simulink model "SW_8"  (R2013b)
settings: Solver=ode45  StartTime=0.0  StopTime=128  RelTol=1e-3
values from neighbouring files (symbols this model uses):
  const_val_lenqs = Nq-1    [confSim.m]    (also in preS_confSim.m)
  g = 1    [confSim.m]
  MiS = -5    [confSim.m]
  MS = 5    [confSim.m]
  nb_counter = ceil(log2(Ns))    [confSim.m]    (also in preS_confSim.m)
  NBitsScoreBus = 10    [confSim.m]    (also in preS_confSim.m)
  Nq = length(qCode)    [confSim.m]    (also in preS_confSim.m)
  Ns = length(sCode)    [confSim.m]    (also in preS_confSim.m)
  qCode = base2dec(q,Base)    [confSim.m]
  sCode = base2dec(s,Base)    [confSim.m]
  SMR_len = Nq*3    [confSim.m]    (also in preS_confSim.m)
libraries: xbsIndex_r4 x1212
(part 7 of 7)

== system SW_8/Subsystem/Subsystem4/P1_HW0/Max1 ==
  (i-1,j) : Inport
  (i,j-1) : Inport  Port=2
  (i-1,j-1) : Inport  Port=3
  Concat : xbsIndex_r4/Concat  num_inputs=2  dbl_ovrd=off  block_type=concat
  Constant4 : xbsIndex_r4/Constant  const=0  gui_display_data_type=Fixed-point  arith_type=Unsigned  n_bits=k  bin_pt=kbp  preci_type=Single  exp_width=8  frac_width=24  explicit_period=on  period=Ts  equ=P=C  opselect=C  inp2=PCIN>>17  opr=+  inp1=P  carry=CIN  dbl_ovrd=off  block_type=constant
  Convert1 : xbsIndex_r4/Convert  gui_display_data_type=Fixed-point  arith_type=Unsigned  n_bits=k  bin_pt=0  float_type=Single  exp_bits=8  fraction_bits=24  quantization=Truncate  overflow=Wrap  en=off  latency=c0  dbl_ovrd=off  pipeline=off  block_type=convert
  Convert3 : xbsIndex_r4/Convert  gui_display_data_type=Fixed-point  arith_type=Unsigned  n_bits=NBitsCalcInt  bin_pt=0  float_type=Single  exp_bits=8  fraction_bits=24  quantization=Truncate  overflow=Wrap  en=off  latency=c0  dbl_ovrd=off  pipeline=off  block_type=convert
  Mux : xbsIndex_r4/Mux  inputs=2  en=off  latency=mft  precision=User Defined  arith_type="Signed  (2's comp)"  n_bits=NBitsCalcInt  bin_pt=0  quantization=Truncate  overflow=Wrap  dbl_ovrd=off  block_type=mux
  Mux1 : xbsIndex_r4/Mux  inputs=2  en=off  latency=mft  precision=User Defined  arith_type=Unsigned  n_bits=nb_bool  bin_pt=0  quantization=Truncate  overflow=Wrap  dbl_ovrd=off  block_type=mux
  Mux2 : xbsIndex_r4/Mux  inputs=2  en=off  latency=mft  precision=User Defined  arith_type="Signed  (2's comp)"  n_bits=NBitsCalcInt  bin_pt=0  quantization=Truncate  overflow=Wrap  dbl_ovrd=off  block_type=mux
  Mux6 : xbsIndex_r4/Mux  inputs=2  en=off  latency=mft  precision=User Defined  arith_type="Signed  (2's comp)"  n_bits=NBitsCalcInt  bin_pt=0  quantization=Truncate  overflow=Wrap  dbl_ovrd=off  block_type=mux
  Relational : xbsIndex_r4/Relational  mode=a>b  en=off  latency=r0  dbl_ovrd=off  block_type=relational
  Relational1 : xbsIndex_r4/Relational  mode=a>b  en=off  latency=r0  dbl_ovrd=off  block_type=relational
  Relational3 : xbsIndex_r4/Relational  mode=a>b  en=off  latency=r0  dbl_ovrd=off  block_type=relational
  ind : Outport  InitialOutput=0
  value : Outport  Port=2  InitialOutput=0
  wires:
  Relational/1 -> Mux1/2, Mux/1
  (i-1,j)/1 -> Relational/1, Mux/3
  Constant4/1 -> Mux/2, Relational/2
  Mux/1 -> Mux2/2, Relational1/2  "MS(q_j,s(n))"
  Mux6/1 -> Mux2/3, Relational1/1
  Relational1/1 -> Concat/1, Mux1/1, Mux2/1
  Mux2/1 -> Convert3/1
  Concat/1 -> Convert1/1
  Relational3/1 -> Mux1/3, Mux6/1
  (i,j-1)/1 -> Mux6/3, Relational3/1
  (i-1,j-1)/1 -> Mux6/2, Relational3/2
  Mux1/1 -> Concat/2
  Convert3/1 -> value/1
  Convert1/1 -> ind/1

== system SW_8/Subsystem/Subsystem4/seq_switch/U>U//z ==
  In1 : Inport
  reset : Inport  Port=2
  Convert1 : xbsIndex_r4/Convert  gui_display_data_type=Fixed-point  arith_type=Unsigned  n_bits=nb_bool  bin_pt=0  float_type=Single  exp_bits=8  fraction_bits=24  quantization=Truncate  overflow=Wrap  en=off  latency=c0  dbl_ovrd=off  pipeline=off  block_type=convert
  R_Nq6 : xbsIndex_r4/Register  init=0  rst=on  en=off  dbl_ovrd=off  block_type=register
  Relational2 : xbsIndex_r4/Relational  mode=a>b  en=off  latency=r0  dbl_ovrd=off  block_type=relational
  Out1 : Outport
  wires:
  Convert1/1 -> R_Nq6/1, Relational2/1
  Relational2/1 -> Out1/1
  R_Nq6/1 -> Relational2/2
  In1/1 -> Convert1/1
  reset/1 -> R_Nq6/2

== system SW_8/Subsystem/Subsystem5/Backtracking_final/Subsystem ==
  i(n-1) : Inport
  D(n) : Inport  Port=2
  AddSub : xbsIndex_r4/AddSub  mode=Subtraction  use_carryin=off  use_carryout=off  en=off  latency=as0  precision=User Defined  arith_type=Unsigned  n_bits=NBitsCalcInt  bin_pt=0  quantization=Truncate  overflow=Wrap  dbl_ovrd=off  use_behavioral_HDL=off  hw_selection=Fabric  pipelined=off  block_type=addsub
  Const_0_2 : xbsIndex_r4/Constant  const=0  gui_display_data_type=Fixed-point  arith_type=Unsigned  n_bits=nb_bool  bin_pt=0  preci_type=Single  exp_width=8  frac_width=24  explicit_period=on  period=Ts  equ=P=C  opselect=C  inp2=PCIN>>17  opr=+  inp1=P  carry=CIN  dbl_ovrd=off  block_type=constant
  Const_1_2 : xbsIndex_r4/Constant  const=1  gui_display_data_type=Fixed-point  arith_type=Unsigned  n_bits=1  bin_pt=0  preci_type=Single  exp_width=8  frac_width=24  explicit_period=on  period=Ts  equ=P=C  opselect=C  inp2=PCIN>>17  opr=+  inp1=P  carry=CIN  dbl_ovrd=off  block_type=constant
  Convert1 : xbsIndex_r4/Convert  gui_display_data_type=Fixed-point  arith_type=Unsigned  n_bits=k  bin_pt=0  float_type=Single  exp_bits=8  fraction_bits=24  quantization=Truncate  overflow=Wrap  en=off  latency=c0  dbl_ovrd=off  pipeline=off  block_type=convert
  Convert2 : xbsIndex_r4/Convert  gui_display_data_type=Fixed-point  arith_type=Unsigned  n_bits=counter_num_b  bin_pt=0  float_type=Single  exp_bits=8  fraction_bits=24  quantization=Truncate  overflow=Wrap  en=off  latency=c0  dbl_ovrd=off  pipeline=off  block_type=convert
  Convert3 : xbsIndex_r4/Convert  gui_display_data_type=Fixed-point  arith_type=Unsigned  n_bits=counter_num_b  bin_pt=0  float_type=Single  exp_bits=8  fraction_bits=24  quantization=Truncate  overflow=Wrap  en=off  latency=c0  dbl_ovrd=off  pipeline=off  block_type=convert
  Mux7 : xbsIndex_r4/Mux  inputs=4  en=off  latency=mft  precision=User Defined  arith_type=Unsigned  n_bits=counter_num_b  bin_pt=0  quantization=Truncate  overflow=Wrap  dbl_ovrd=off  block_type=mux
  Mux8 : xbsIndex_r4/Mux  inputs=2  en=off  latency=mft  precision=User Defined  arith_type=Unsigned  n_bits=counter_num_b  bin_pt=0  quantization=Truncate  overflow=Wrap  dbl_ovrd=off  block_type=mux
  Relational2 : xbsIndex_r4/Relational  mode=a<b  en=off  latency=r0  dbl_ovrd=off  block_type=relational
  i(n) : Outport
  StopTBC1 : Outport  Port=2
  wires:
  Convert3/1 -> i(n)/1
  Convert1/1 -> Mux7/1
  Convert2/1 -> Mux7/5, AddSub/1
  Const_1_2/1 -> AddSub/2
  Mux7/1 -> Relational2/1, Mux8/2
  AddSub/1 -> Mux7/3, Mux7/4
  Relational2/1 -> Mux8/1, StopTBC1/1
  Mux8/1 -> Convert3/1
  i(n-1)/1 -> Convert2/1
  D(n)/1 -> Convert1/1
  Const_0_2/1 -> Mux7/2, Relational2/2, Mux8/3

== system SW_8/Subsystem/Subsystem5/Backtracking_final/hi_lo_cast22 ==
  In1 : Inport
  Concat : xbsIndex_r4/Concat  num_inputs=2  dbl_ovrd=off  block_type=concat
  Convert13 : xbsIndex_r4/Convert  gui_display_data_type=Fixed-point  arith_type=Unsigned  n_bits=k  bin_pt=0  float_type=Single  exp_bits=8  fraction_bits=24  quantization=Truncate  overflow=Wrap  en=off  latency=c0  dbl_ovrd=off  pipeline=off  block_type=convert
  Out1 : Outport
  wires:
  In1/1 -> Concat/1, Concat/2
  Concat/1 -> Convert13/1
  Convert13/1 -> Out1/1

== system SW_8/Subsystem/Subsystem5/P1_HW0/Match and Mismtach Score ==
  q_j : Inport
  s(n) : Inport  Port=2
  MS : Inport  Port=3
  MiS : Inport  Port=4
  Mux : xbsIndex_r4/Mux  inputs=2  en=off  latency=mft  precision=User Defined  arith_type="Signed  (2's comp)"  n_bits=NBitsK  bin_pt=0  quantization=Truncate  overflow=Wrap  dbl_ovrd=off  block_type=mux
  Relational : xbsIndex_r4/Relational  mode=a=b  en=off  latency=r0  dbl_ovrd=off  block_type=relational
  MS(q_j,s(n)) : Outport
  wires:
  MiS/1 -> Mux/2
  MS/1 -> Mux/3
  Relational/1 -> Mux/1
  s(n)/1 -> Relational/2
  Mux/1 -> MS(q_j,s(n))/1  "MS(q_j,s(n))"
  q_j/1 -> Relational/1

== system SW_8/Subsystem/Subsystem5/P1_HW0/Max1 ==
  (i-1,j) : Inport
  (i,j-1) : Inport  Port=2
  (i-1,j-1) : Inport  Port=3
  Concat : xbsIndex_r4/Concat  num_inputs=2  dbl_ovrd=off  block_type=concat
  Constant4 : xbsIndex_r4/Constant  const=0  gui_display_data_type=Fixed-point  arith_type=Unsigned  n_bits=k  bin_pt=kbp  preci_type=Single  exp_width=8  frac_width=24  explicit_period=on  period=Ts  equ=P=C  opselect=C  inp2=PCIN>>17  opr=+  inp1=P  carry=CIN  dbl_ovrd=off  block_type=constant
  Convert1 : xbsIndex_r4/Convert  gui_display_data_type=Fixed-point  arith_type=Unsigned  n_bits=k  bin_pt=0  float_type=Single  exp_bits=8  fraction_bits=24  quantization=Truncate  overflow=Wrap  en=off  latency=c0  dbl_ovrd=off  pipeline=off  block_type=convert
  Convert3 : xbsIndex_r4/Convert  gui_display_data_type=Fixed-point  arith_type=Unsigned  n_bits=NBitsCalcInt  bin_pt=0  float_type=Single  exp_bits=8  fraction_bits=24  quantization=Truncate  overflow=Wrap  en=off  latency=c0  dbl_ovrd=off  pipeline=off  block_type=convert
  Mux : xbsIndex_r4/Mux  inputs=2  en=off  latency=mft  precision=User Defined  arith_type="Signed  (2's comp)"  n_bits=NBitsCalcInt  bin_pt=0  quantization=Truncate  overflow=Wrap  dbl_ovrd=off  block_type=mux
  Mux1 : xbsIndex_r4/Mux  inputs=2  en=off  latency=mft  precision=User Defined  arith_type=Unsigned  n_bits=nb_bool  bin_pt=0  quantization=Truncate  overflow=Wrap  dbl_ovrd=off  block_type=mux
  Mux2 : xbsIndex_r4/Mux  inputs=2  en=off  latency=mft  precision=User Defined  arith_type="Signed  (2's comp)"  n_bits=NBitsCalcInt  bin_pt=0  quantization=Truncate  overflow=Wrap  dbl_ovrd=off  block_type=mux
  Mux6 : xbsIndex_r4/Mux  inputs=2  en=off  latency=mft  precision=User Defined  arith_type="Signed  (2's comp)"  n_bits=NBitsCalcInt  bin_pt=0  quantization=Truncate  overflow=Wrap  dbl_ovrd=off  block_type=mux
  Relational : xbsIndex_r4/Relational  mode=a>b  en=off  latency=r0  dbl_ovrd=off  block_type=relational
  Relational1 : xbsIndex_r4/Relational  mode=a>b  en=off  latency=r0  dbl_ovrd=off  block_type=relational
  Relational3 : xbsIndex_r4/Relational  mode=a>b  en=off  latency=r0  dbl_ovrd=off  block_type=relational
  ind : Outport  InitialOutput=0
  value : Outport  Port=2  InitialOutput=0
  wires:
  Relational/1 -> Mux1/2, Mux/1
  (i-1,j)/1 -> Relational/1, Mux/3
  Constant4/1 -> Mux/2, Relational/2
  Mux/1 -> Mux2/2, Relational1/2  "MS(q_j,s(n))"
  Mux6/1 -> Mux2/3, Relational1/1
  Relational1/1 -> Concat/1, Mux1/1, Mux2/1
  Mux2/1 -> Convert3/1
  Concat/1 -> Convert1/1
  Relational3/1 -> Mux1/3, Mux6/1
  (i,j-1)/1 -> Mux6/3, Relational3/1
  (i-1,j-1)/1 -> Mux6/2, Relational3/2
  Mux1/1 -> Concat/2
  Convert3/1 -> value/1
  Convert1/1 -> ind/1

== system SW_8/Subsystem/Subsystem5/seq_switch/U>U//z ==
  In1 : Inport
  reset : Inport  Port=2
  Convert1 : xbsIndex_r4/Convert  gui_display_data_type=Fixed-point  arith_type=Unsigned  n_bits=nb_bool  bin_pt=0  float_type=Single  exp_bits=8  fraction_bits=24  quantization=Truncate  overflow=Wrap  en=off  latency=c0  dbl_ovrd=off  pipeline=off  block_type=convert
  R_Nq6 : xbsIndex_r4/Register  init=0  rst=on  en=off  dbl_ovrd=off  block_type=register
  Relational2 : xbsIndex_r4/Relational  mode=a>b  en=off  latency=r0  dbl_ovrd=off  block_type=relational
  Out1 : Outport
  wires:
  Convert1/1 -> R_Nq6/1, Relational2/1
  Relational2/1 -> Out1/1
  R_Nq6/1 -> Relational2/2
  In1/1 -> Convert1/1
  reset/1 -> R_Nq6/2

== system SW_8/Subsystem/Subsystem6/Backtracking_final/Subsystem ==
  i(n-1) : Inport
  D(n) : Inport  Port=2
  AddSub : xbsIndex_r4/AddSub  mode=Subtraction  use_carryin=off  use_carryout=off  en=off  latency=as0  precision=User Defined  arith_type=Unsigned  n_bits=NBitsCalcInt  bin_pt=0  quantization=Truncate  overflow=Wrap  dbl_ovrd=off  use_behavioral_HDL=off  hw_selection=Fabric  pipelined=off  block_type=addsub
  Const_0_2 : xbsIndex_r4/Constant  const=0  gui_display_data_type=Fixed-point  arith_type=Unsigned  n_bits=nb_bool  bin_pt=0  preci_type=Single  exp_width=8  frac_width=24  explicit_period=on  period=Ts  equ=P=C  opselect=C  inp2=PCIN>>17  opr=+  inp1=P  carry=CIN  dbl_ovrd=off  block_type=constant
  Const_1_2 : xbsIndex_r4/Constant  const=1  gui_display_data_type=Fixed-point  arith_type=Unsigned  n_bits=1  bin_pt=0  preci_type=Single  exp_width=8  frac_width=24  explicit_period=on  period=Ts  equ=P=C  opselect=C  inp2=PCIN>>17  opr=+  inp1=P  carry=CIN  dbl_ovrd=off  block_type=constant
  Convert1 : xbsIndex_r4/Convert  gui_display_data_type=Fixed-point  arith_type=Unsigned  n_bits=k  bin_pt=0  float_type=Single  exp_bits=8  fraction_bits=24  quantization=Truncate  overflow=Wrap  en=off  latency=c0  dbl_ovrd=off  pipeline=off  block_type=convert
  Convert2 : xbsIndex_r4/Convert  gui_display_data_type=Fixed-point  arith_type=Unsigned  n_bits=counter_num_b  bin_pt=0  float_type=Single  exp_bits=8  fraction_bits=24  quantization=Truncate  overflow=Wrap  en=off  latency=c0  dbl_ovrd=off  pipeline=off  block_type=convert
  Convert3 : xbsIndex_r4/Convert  gui_display_data_type=Fixed-point  arith_type=Unsigned  n_bits=counter_num_b  bin_pt=0  float_type=Single  exp_bits=8  fraction_bits=24  quantization=Truncate  overflow=Wrap  en=off  latency=c0  dbl_ovrd=off  pipeline=off  block_type=convert
  Mux7 : xbsIndex_r4/Mux  inputs=4  en=off  latency=mft  precision=User Defined  arith_type=Unsigned  n_bits=counter_num_b  bin_pt=0  quantization=Truncate  overflow=Wrap  dbl_ovrd=off  block_type=mux
  Mux8 : xbsIndex_r4/Mux  inputs=2  en=off  latency=mft  precision=User Defined  arith_type=Unsigned  n_bits=counter_num_b  bin_pt=0  quantization=Truncate  overflow=Wrap  dbl_ovrd=off  block_type=mux
  Relational2 : xbsIndex_r4/Relational  mode=a<b  en=off  latency=r0  dbl_ovrd=off  block_type=relational
  i(n) : Outport
  StopTBC1 : Outport  Port=2
  wires:
  Convert3/1 -> i(n)/1
  Convert1/1 -> Mux7/1
  Convert2/1 -> Mux7/5, AddSub/1
  Const_1_2/1 -> AddSub/2
  Mux7/1 -> Relational2/1, Mux8/2
  AddSub/1 -> Mux7/3, Mux7/4
  Relational2/1 -> Mux8/1, StopTBC1/1
  Mux8/1 -> Convert3/1
  i(n-1)/1 -> Convert2/1
  D(n)/1 -> Convert1/1
  Const_0_2/1 -> Mux7/2, Relational2/2, Mux8/3

== system SW_8/Subsystem/Subsystem6/Backtracking_final/hi_lo_cast22 ==
  In1 : Inport
  Concat : xbsIndex_r4/Concat  num_inputs=2  dbl_ovrd=off  block_type=concat
  Convert13 : xbsIndex_r4/Convert  gui_display_data_type=Fixed-point  arith_type=Unsigned  n_bits=k  bin_pt=0  float_type=Single  exp_bits=8  fraction_bits=24  quantization=Truncate  overflow=Wrap  en=off  latency=c0  dbl_ovrd=off  pipeline=off  block_type=convert
  Out1 : Outport
  wires:
  In1/1 -> Concat/1, Concat/2
  Concat/1 -> Convert13/1
  Convert13/1 -> Out1/1

== system SW_8/Subsystem/Subsystem6/P1_HW0/Match and Mismtach Score ==
  q_j : Inport
  s(n) : Inport  Port=2
  MS : Inport  Port=3
  MiS : Inport  Port=4
  Mux : xbsIndex_r4/Mux  inputs=2  en=off  latency=mft  precision=User Defined  arith_type="Signed  (2's comp)"  n_bits=NBitsK  bin_pt=0  quantization=Truncate  overflow=Wrap  dbl_ovrd=off  block_type=mux
  Relational : xbsIndex_r4/Relational  mode=a=b  en=off  latency=r0  dbl_ovrd=off  block_type=relational
  MS(q_j,s(n)) : Outport
  wires:
  MiS/1 -> Mux/2
  MS/1 -> Mux/3
  Relational/1 -> Mux/1
  s(n)/1 -> Relational/2
  Mux/1 -> MS(q_j,s(n))/1  "MS(q_j,s(n))"
  q_j/1 -> Relational/1

== system SW_8/Subsystem/Subsystem6/P1_HW0/Max1 ==
  (i-1,j) : Inport
  (i,j-1) : Inport  Port=2
  (i-1,j-1) : Inport  Port=3
  Concat : xbsIndex_r4/Concat  num_inputs=2  dbl_ovrd=off  block_type=concat
  Constant4 : xbsIndex_r4/Constant  const=0  gui_display_data_type=Fixed-point  arith_type=Unsigned  n_bits=k  bin_pt=kbp  preci_type=Single  exp_width=8  frac_width=24  explicit_period=on  period=Ts  equ=P=C  opselect=C  inp2=PCIN>>17  opr=+  inp1=P  carry=CIN  dbl_ovrd=off  block_type=constant
  Convert1 : xbsIndex_r4/Convert  gui_display_data_type=Fixed-point  arith_type=Unsigned  n_bits=k  bin_pt=0  float_type=Single  exp_bits=8  fraction_bits=24  quantization=Truncate  overflow=Wrap  en=off  latency=c0  dbl_ovrd=off  pipeline=off  block_type=convert
  Convert3 : xbsIndex_r4/Convert  gui_display_data_type=Fixed-point  arith_type=Unsigned  n_bits=NBitsCalcInt  bin_pt=0  float_type=Single  exp_bits=8  fraction_bits=24  quantization=Truncate  overflow=Wrap  en=off  latency=c0  dbl_ovrd=off  pipeline=off  block_type=convert
  Mux : xbsIndex_r4/Mux  inputs=2  en=off  latency=mft  precision=User Defined  arith_type="Signed  (2's comp)"  n_bits=NBitsCalcInt  bin_pt=0  quantization=Truncate  overflow=Wrap  dbl_ovrd=off  block_type=mux
  Mux1 : xbsIndex_r4/Mux  inputs=2  en=off  latency=mft  precision=User Defined  arith_type=Unsigned  n_bits=nb_bool  bin_pt=0  quantization=Truncate  overflow=Wrap  dbl_ovrd=off  block_type=mux
  Mux2 : xbsIndex_r4/Mux  inputs=2  en=off  latency=mft  precision=User Defined  arith_type="Signed  (2's comp)"  n_bits=NBitsCalcInt  bin_pt=0  quantization=Truncate  overflow=Wrap  dbl_ovrd=off  block_type=mux
  Mux6 : xbsIndex_r4/Mux  inputs=2  en=off  latency=mft  precision=User Defined  arith_type="Signed  (2's comp)"  n_bits=NBitsCalcInt  bin_pt=0  quantization=Truncate  overflow=Wrap  dbl_ovrd=off  block_type=mux
  Relational : xbsIndex_r4/Relational  mode=a>b  en=off  latency=r0  dbl_ovrd=off  block_type=relational
  Relational1 : xbsIndex_r4/Relational  mode=a>b  en=off  latency=r0  dbl_ovrd=off  block_type=relational
  Relational3 : xbsIndex_r4/Relational  mode=a>b  en=off  latency=r0  dbl_ovrd=off  block_type=relational
  ind : Outport  InitialOutput=0
  value : Outport  Port=2  InitialOutput=0
  wires:
  Relational/1 -> Mux1/2, Mux/1
  (i-1,j)/1 -> Relational/1, Mux/3
  Constant4/1 -> Mux/2, Relational/2
  Mux/1 -> Mux2/2, Relational1/2  "MS(q_j,s(n))"
  Mux6/1 -> Mux2/3, Relational1/1
  Relational1/1 -> Concat/1, Mux1/1, Mux2/1
  Mux2/1 -> Convert3/1
  Concat/1 -> Convert1/1
  Relational3/1 -> Mux1/3, Mux6/1
  (i,j-1)/1 -> Mux6/3, Relational3/1
  (i-1,j-1)/1 -> Mux6/2, Relational3/2
  Mux1/1 -> Concat/2
  Convert3/1 -> value/1
  Convert1/1 -> ind/1

== system SW_8/Subsystem/Subsystem6/seq_switch/U>U//z ==
  In1 : Inport
  reset : Inport  Port=2
  Convert1 : xbsIndex_r4/Convert  gui_display_data_type=Fixed-point  arith_type=Unsigned  n_bits=nb_bool  bin_pt=0  float_type=Single  exp_bits=8  fraction_bits=24  quantization=Truncate  overflow=Wrap  en=off  latency=c0  dbl_ovrd=off  pipeline=off  block_type=convert
  R_Nq6 : xbsIndex_r4/Register  init=0  rst=on  en=off  dbl_ovrd=off  block_type=register
  Relational2 : xbsIndex_r4/Relational  mode=a>b  en=off  latency=r0  dbl_ovrd=off  block_type=relational
  Out1 : Outport
  wires:
  Convert1/1 -> R_Nq6/1, Relational2/1
  Relational2/1 -> Out1/1
  R_Nq6/1 -> Relational2/2
  In1/1 -> Convert1/1
  reset/1 -> R_Nq6/2

== system SW_8/Subsystem/Subsystem7/Backtracking_final/Subsystem ==
  i(n-1) : Inport
  D(n) : Inport  Port=2
  AddSub : xbsIndex_r4/AddSub  mode=Subtraction  use_carryin=off  use_carryout=off  en=off  latency=as0  precision=User Defined  arith_type=Unsigned  n_bits=NBitsCalcInt  bin_pt=0  quantization=Truncate  overflow=Wrap  dbl_ovrd=off  use_behavioral_HDL=off  hw_selection=Fabric  pipelined=off  block_type=addsub
  Const_0_2 : xbsIndex_r4/Constant  const=0  gui_display_data_type=Fixed-point  arith_type=Unsigned  n_bits=nb_bool  bin_pt=0  preci_type=Single  exp_width=8  frac_width=24  explicit_period=on  period=Ts  equ=P=C  opselect=C  inp2=PCIN>>17  opr=+  inp1=P  carry=CIN  dbl_ovrd=off  block_type=constant
  Const_1_2 : xbsIndex_r4/Constant  const=1  gui_display_data_type=Fixed-point  arith_type=Unsigned  n_bits=1  bin_pt=0  preci_type=Single  exp_width=8  frac_width=24  explicit_period=on  period=Ts  equ=P=C  opselect=C  inp2=PCIN>>17  opr=+  inp1=P  carry=CIN  dbl_ovrd=off  block_type=constant
  Convert1 : xbsIndex_r4/Convert  gui_display_data_type=Fixed-point  arith_type=Unsigned  n_bits=k  bin_pt=0  float_type=Single  exp_bits=8  fraction_bits=24  quantization=Truncate  overflow=Wrap  en=off  latency=c0  dbl_ovrd=off  pipeline=off  block_type=convert
  Convert2 : xbsIndex_r4/Convert  gui_display_data_type=Fixed-point  arith_type=Unsigned  n_bits=counter_num_b  bin_pt=0  float_type=Single  exp_bits=8  fraction_bits=24  quantization=Truncate  overflow=Wrap  en=off  latency=c0  dbl_ovrd=off  pipeline=off  block_type=convert
  Convert3 : xbsIndex_r4/Convert  gui_display_data_type=Fixed-point  arith_type=Unsigned  n_bits=counter_num_b  bin_pt=0  float_type=Single  exp_bits=8  fraction_bits=24  quantization=Truncate  overflow=Wrap  en=off  latency=c0  dbl_ovrd=off  pipeline=off  block_type=convert
  Mux7 : xbsIndex_r4/Mux  inputs=4  en=off  latency=mft  precision=User Defined  arith_type=Unsigned  n_bits=counter_num_b  bin_pt=0  quantization=Truncate  overflow=Wrap  dbl_ovrd=off  block_type=mux
  Mux8 : xbsIndex_r4/Mux  inputs=2  en=off  latency=mft  precision=User Defined  arith_type=Unsigned  n_bits=counter_num_b  bin_pt=0  quantization=Truncate  overflow=Wrap  dbl_ovrd=off  block_type=mux
  Relational2 : xbsIndex_r4/Relational  mode=a<b  en=off  latency=r0  dbl_ovrd=off  block_type=relational
  i(n) : Outport
  StopTBC1 : Outport  Port=2
  wires:
  Convert3/1 -> i(n)/1
  Convert1/1 -> Mux7/1
  Convert2/1 -> Mux7/5, AddSub/1
  Const_1_2/1 -> AddSub/2
  Mux7/1 -> Relational2/1, Mux8/2
  AddSub/1 -> Mux7/3, Mux7/4
  Relational2/1 -> Mux8/1, StopTBC1/1
  Mux8/1 -> Convert3/1
  i(n-1)/1 -> Convert2/1
  D(n)/1 -> Convert1/1
  Const_0_2/1 -> Mux7/2, Relational2/2, Mux8/3

== system SW_8/Subsystem/Subsystem7/Backtracking_final/hi_lo_cast22 ==
  In1 : Inport
  Concat : xbsIndex_r4/Concat  num_inputs=2  dbl_ovrd=off  block_type=concat
  Convert13 : xbsIndex_r4/Convert  gui_display_data_type=Fixed-point  arith_type=Unsigned  n_bits=k  bin_pt=0  float_type=Single  exp_bits=8  fraction_bits=24  quantization=Truncate  overflow=Wrap  en=off  latency=c0  dbl_ovrd=off  pipeline=off  block_type=convert
  Out1 : Outport
  wires:
  In1/1 -> Concat/1, Concat/2
  Concat/1 -> Convert13/1
  Convert13/1 -> Out1/1

== system SW_8/Subsystem/Subsystem7/P1_HW0/Match and Mismtach Score ==
  q_j : Inport
  s(n) : Inport  Port=2
  MS : Inport  Port=3
  MiS : Inport  Port=4
  Mux : xbsIndex_r4/Mux  inputs=2  en=off  latency=mft  precision=User Defined  arith_type="Signed  (2's comp)"  n_bits=NBitsK  bin_pt=0  quantization=Truncate  overflow=Wrap  dbl_ovrd=off  block_type=mux
  Relational : xbsIndex_r4/Relational  mode=a=b  en=off  latency=r0  dbl_ovrd=off  block_type=relational
  MS(q_j,s(n)) : Outport
  wires:
  MiS/1 -> Mux/2
  MS/1 -> Mux/3
  Relational/1 -> Mux/1
  s(n)/1 -> Relational/2
  Mux/1 -> MS(q_j,s(n))/1  "MS(q_j,s(n))"
  q_j/1 -> Relational/1

== system SW_8/Subsystem/Subsystem7/P1_HW0/Max1 ==
  (i-1,j) : Inport
  (i,j-1) : Inport  Port=2
  (i-1,j-1) : Inport  Port=3
  Concat : xbsIndex_r4/Concat  num_inputs=2  dbl_ovrd=off  block_type=concat
  Constant4 : xbsIndex_r4/Constant  const=0  gui_display_data_type=Fixed-point  arith_type=Unsigned  n_bits=k  bin_pt=kbp  preci_type=Single  exp_width=8  frac_width=24  explicit_period=on  period=Ts  equ=P=C  opselect=C  inp2=PCIN>>17  opr=+  inp1=P  carry=CIN  dbl_ovrd=off  block_type=constant
  Convert1 : xbsIndex_r4/Convert  gui_display_data_type=Fixed-point  arith_type=Unsigned  n_bits=k  bin_pt=0  float_type=Single  exp_bits=8  fraction_bits=24  quantization=Truncate  overflow=Wrap  en=off  latency=c0  dbl_ovrd=off  pipeline=off  block_type=convert
  Convert3 : xbsIndex_r4/Convert  gui_display_data_type=Fixed-point  arith_type=Unsigned  n_bits=NBitsCalcInt  bin_pt=0  float_type=Single  exp_bits=8  fraction_bits=24  quantization=Truncate  overflow=Wrap  en=off  latency=c0  dbl_ovrd=off  pipeline=off  block_type=convert
  Mux : xbsIndex_r4/Mux  inputs=2  en=off  latency=mft  precision=User Defined  arith_type="Signed  (2's comp)"  n_bits=NBitsCalcInt  bin_pt=0  quantization=Truncate  overflow=Wrap  dbl_ovrd=off  block_type=mux
  Mux1 : xbsIndex_r4/Mux  inputs=2  en=off  latency=mft  precision=User Defined  arith_type=Unsigned  n_bits=nb_bool  bin_pt=0  quantization=Truncate  overflow=Wrap  dbl_ovrd=off  block_type=mux
  Mux2 : xbsIndex_r4/Mux  inputs=2  en=off  latency=mft  precision=User Defined  arith_type="Signed  (2's comp)"  n_bits=NBitsCalcInt  bin_pt=0  quantization=Truncate  overflow=Wrap  dbl_ovrd=off  block_type=mux
  Mux6 : xbsIndex_r4/Mux  inputs=2  en=off  latency=mft  precision=User Defined  arith_type="Signed  (2's comp)"  n_bits=NBitsCalcInt  bin_pt=0  quantization=Truncate  overflow=Wrap  dbl_ovrd=off  block_type=mux
  Relational : xbsIndex_r4/Relational  mode=a>b  en=off  latency=r0  dbl_ovrd=off  block_type=relational
  Relational1 : xbsIndex_r4/Relational  mode=a>b  en=off  latency=r0  dbl_ovrd=off  block_type=relational
  Relational3 : xbsIndex_r4/Relational  mode=a>b  en=off  latency=r0  dbl_ovrd=off  block_type=relational
  ind : Outport  InitialOutput=0
  value : Outport  Port=2  InitialOutput=0
  wires:
  Relational/1 -> Mux1/2, Mux/1
  (i-1,j)/1 -> Relational/1, Mux/3
  Constant4/1 -> Mux/2, Relational/2
  Mux/1 -> Mux2/2, Relational1/2  "MS(q_j,s(n))"
  Mux6/1 -> Mux2/3, Relational1/1
  Relational1/1 -> Concat/1, Mux1/1, Mux2/1
  Mux2/1 -> Convert3/1
  Concat/1 -> Convert1/1
  Relational3/1 -> Mux1/3, Mux6/1
  (i,j-1)/1 -> Mux6/3, Relational3/1
  (i-1,j-1)/1 -> Mux6/2, Relational3/2
  Mux1/1 -> Concat/2
  Convert3/1 -> value/1
  Convert1/1 -> ind/1

== system SW_8/Subsystem/Subsystem7/seq_switch/U>U//z ==
  In1 : Inport
  reset : Inport  Port=2
  Convert1 : xbsIndex_r4/Convert  gui_display_data_type=Fixed-point  arith_type=Unsigned  n_bits=nb_bool  bin_pt=0  float_type=Single  exp_bits=8  fraction_bits=24  quantization=Truncate  overflow=Wrap  en=off  latency=c0  dbl_ovrd=off  pipeline=off  block_type=convert
  R_Nq6 : xbsIndex_r4/Register  init=0  rst=on  en=off  dbl_ovrd=off  block_type=register
  Relational2 : xbsIndex_r4/Relational  mode=a>b  en=off  latency=r0  dbl_ovrd=off  block_type=relational
  Out1 : Outport
  wires:
  Convert1/1 -> R_Nq6/1, Relational2/1
  Relational2/1 -> Out1/1
  R_Nq6/1 -> Relational2/2
  In1/1 -> Convert1/1
  reset/1 -> R_Nq6/2
